simulink model "domin_trend"  (Simulink 7.9)
settings: Solver=ode45  StartTime=0.0  StopTime=600  RelTol=1e-3
settings Model: Creator=eee  LastModifiedBy=eee

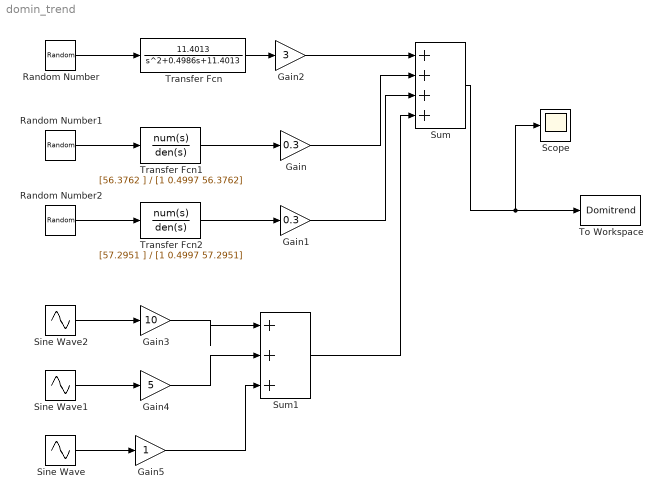
== system domin_trend ==
  Gain : Gain  Gain=0.3
  Gain1 : Gain  Gain=0.3
  Gain2 : Gain  Gain=3
  Gain3 : Gain  Gain=10
  Gain4 : Gain  Gain=5
  Gain5 : Gain
  Random Number : RandomNumber  SampleTime=0.1
  Random Number1 : RandomNumber  SampleTime=0.1
  Random Number2 : RandomNumber  SampleTime=0.1
  Scope : Scope
      settings: TimeRange=500  YMin=-2  YMax=2.5
  Sine Wave : Sin  Frequency=.05  SampleTime=0
  Sine Wave1 : Sin  Frequency=.03  SampleTime=0
  Sine Wave2 : Sin  Frequency=.01  SampleTime=0
  Sum : Sum  Inputs=|++++
  Sum1 : Sum  Inputs=|+++
  To Workspace : ToWorkspace  VariableName=Domitrend  SampleTime=-1
  Transfer Fcn : TransferFcn  Numerator=[11.4013 ]  Denominator=[1 0.4986 11.4013]
  Transfer Fcn1 : TransferFcn  Numerator=[56.3762 ]  Denominator=[1 0.4997 56.3762]
  Transfer Fcn2 : TransferFcn  Numerator=[57.2951 ]  Denominator=[1 0.4997 57.2951]
  wires:
  Random Number/1 -> Transfer Fcn/1
  Random Number1/1 -> Transfer Fcn1/1
  Random Number2/1 -> Transfer Fcn2/1
  Transfer Fcn/1 -> Gain2/1
  Transfer Fcn1/1 -> Gain/1
  Transfer Fcn2/1 -> Gain1/1
  Gain2/1 -> Sum/1
  Gain/1 -> Sum/2
  Gain1/1 -> Sum/3
  Sum/1 -> To Workspace/1, Scope/1
  Sine Wave1/1 -> Gain4/1
  Sine Wave2/1 -> Gain3/1
  Sine Wave/1 -> Gain5/1
  Gain3/1 -> Sum1/1
  Gain4/1 -> Sum1/2
  Gain5/1 -> Sum1/3
  Sum1/1 -> Sum/4
